simulink model "EstimFirstOrder"  (R2021a)
settings: Solver=FixedStepAuto  StartTime=0.0  StopTime=TWindow  FixedStep=Ts  RelTol=1e-3
values from neighbouring files (symbols this model uses):
  N = 1000    [params.m]
  P = conv(Poly1,Poly2)    [params.m]
  Q = [-3 2]    [params.m]
  Ts = 0.001    [params.m]
settings Model: Creator=perruquetti  LastModifiedBy=perruquetti

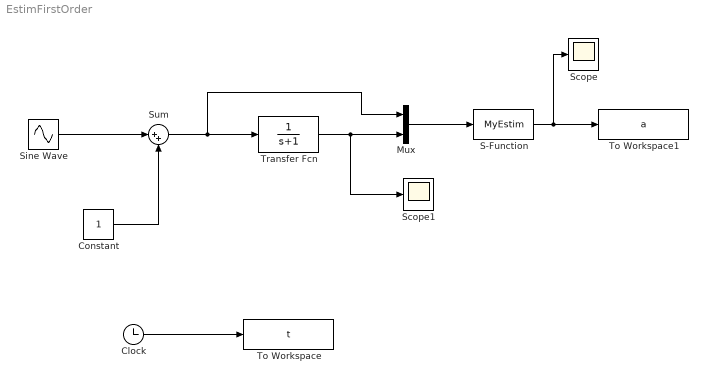
== system EstimFirstOrder ==
  Clock : Clock
  Constant : Constant
  Mux : Mux  Inputs=2
  S-Function : S-Function  FunctionName=MyEstim  Parameters=N,Ts,P,Q  SFunctionDeploymentMode=off  EnableBusSupport=off
  Scope : Scope
  Scope1 : Scope
  Sine Wave : Sin  Frequency=10  SampleTime=0
  Sum : Sum  Inputs=|++
  To Workspace : ToWorkspace  VariableName=t  SampleTime=-1
  To Workspace1 : ToWorkspace  VariableName=a  SampleTime=-1
  Transfer Fcn : TransferFcn  Denominator=[1 1]  ParameterTunability=Unconstrained
  wires:
  Constant/1 -> Sum/2
  Sine Wave/1 -> Sum/1
  Sum/1 -> Mux/1, Transfer Fcn/1
  Clock/1 -> To Workspace/1
  Transfer Fcn/1 -> Scope1/1, Mux/2
  Mux/1 -> S-Function/1
  S-Function/1 -> Scope/1, To Workspace1/1
